simulink model "ieee_6_bus_base_case"  (R2015b)
settings: Solver=FixedStepAuto  StartTime=0.0  StopTime=25  FixedStep=Ts  RelTol=1e-3
values from neighbouring files (symbols this model uses):
  Cbase = 1/(100*pi*Xbase)    (= 1.34217357979e-05)    [ieee_6_bus.m]
  Lbase = Xbase/(100*pi)    (= 0.754903726073)    [ieee_6_bus.m]
  Ts = 1e-5    (= 1e-05)    [ieee_6_bus.m]
  Xbase = (Vbase^2)/Sbase    (= 237.16)    [ieee_6_bus.m]
undefined symbols (not defined in the file or in its folder): loadconnection, startup
libraries: powerlib x153, powerlib_meascontrol x7, sps_avr x4, simulink x1
(part 1 of 2)
settings Model: SimulationMode=accelerator  Creator=Eren  LastModifiedBy=Eren
settings SolverCC: AlgebraicLoopSolver=LineSearch

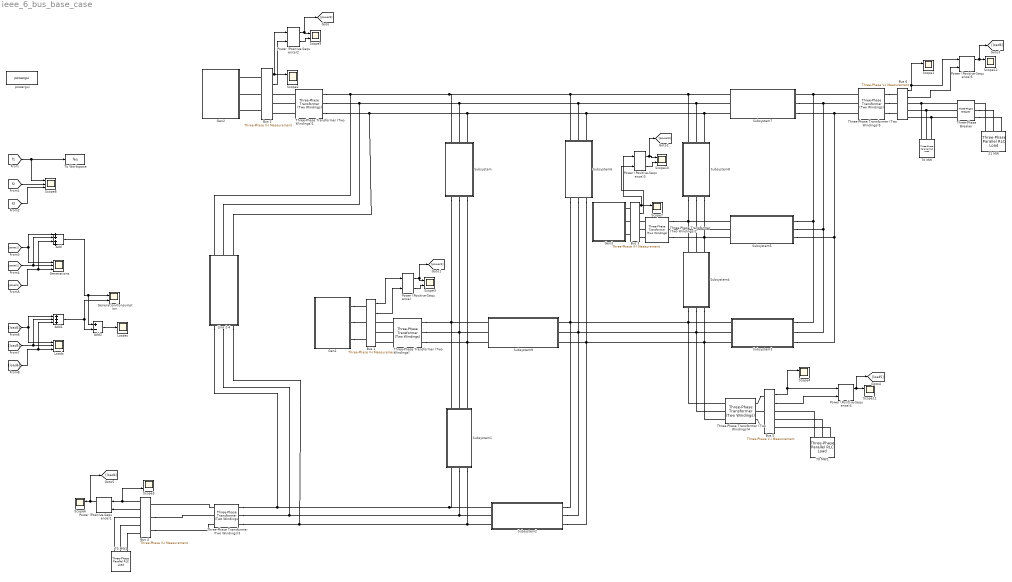
== system ieee_6_bus_base_case ==
  21 MW : powerlib/Elements/Three-Phase Parallel RLC Load  LConnTagsString=A|B|C  Configuration=Y (grounded)  NominalVoltage=690  Vabc=[1e3 1e3 1e3]  Vabcp=[1e3 1e3 1e3]  NominalFrequency=50  UnbalancedPower=off  ActivePower=21e6  InductivePower=0  CapacitivePower=0  Pabc=[10e3 9e3 11e3]  QLabc=[100 90 110]  QCabc=[100 90 110]  Pabcp=[10e3 9e3 11e3]  QLabcp=[100 90 110]  QCabcp=[100 90 110]  Measurements=None  LoadType=constant PQ
  70 MW : powerlib/Elements/Three-Phase Parallel RLC Load  LConnTagsString=A|B|C  Configuration=Y (grounded)  NominalVoltage=690  Vabc=[1e3 1e3 1e3]  Vabcp=[1e3 1e3 1e3]  NominalFrequency=50  UnbalancedPower=off  ActivePower=70e6  InductivePower=70e6  CapacitivePower=0  Pabc=[10e3 9e3 11e3]  QLabc=[100 90 110]  QCabc=[100 90 110]  Pabcp=[10e3 9e3 11e3]  QLabcp=[100 90 110]  QCabcp=[100 90 110]  Measurements=None  LoadType=constant PQ
  70 MW1 : powerlib/Elements/Three-Phase Parallel RLC Load  LConnTagsString=A|B|C  Configuration=Y (grounded)  NominalVoltage=690  Vabc=[1e3 1e3 1e3]  Vabcp=[1e3 1e3 1e3]  NominalFrequency=50  UnbalancedPower=off  ActivePower=70e6  InductivePower=70e6  CapacitivePower=0  Pabc=[10e3 9e3 11e3]  QLabc=[100 90 110]  QCabc=[100 90 110]  Pabcp=[10e3 9e3 11e3]  QLabcp=[100 90 110]  QCabcp=[100 90 110]  Measurements=None  LoadType=constant PQ
  70 MW2 : powerlib/Elements/Three-Phase Parallel RLC Load  LConnTagsString=A|B|C  Configuration=Y (grounded)  NominalVoltage=690  Vabc=[1e3 1e3 1e3]  Vabcp=[1e3 1e3 1e3]  NominalFrequency=50  UnbalancedPower=off  ActivePower=70e6  InductivePower=70e6  CapacitivePower=0  Pabc=[10e3 9e3 11e3]  QLabc=[100 90 110]  QCabc=[100 90 110]  Pabcp=[10e3 9e3 11e3]  QLabcp=[100 90 110]  QCabcp=[100 90 110]  Measurements=None  LoadType=constant PQ
  Add : Sum  Inputs=4
  Add1 : Sum  Inputs=3
  Add2 : Sum  Inputs=+-
  Bus {1..4,6} (5 alike) : powerlib/Measurements/Three-Phase V-I Measurement  VoltageMeasurement=phase-to-ground  SetLabelV=off  LabelV=Vsabc  Vpu=off  VpuLL=on  CurrentMeasurement=yes  SetLabelI=off  LabelI=Isabc  Ipu=off  Pbase=100e6  Vbase=690  OutputType=Complex  PhasorSimulation=off  PSBequivalent=0
  Bus 5 : powerlib/Measurements/Three-Phase V-I Measurement  VoltageMeasurement=phase-to-ground  SetLabelV=off  LabelV=Vsabc  Vpu=off  VpuLL=off  CurrentMeasurement=yes  SetLabelI=off  LabelI=Isabc  Ipu=off  Pbase=100e6  Vbase=690  OutputType=Complex  PhasorSimulation=off  PSBequivalent=0
  Gen1 : Subsystem
  Gen2 : Subsystem
  Gen3 : Subsystem
  Generation/Consumption : Scope  NumInputPorts=2
  Generations : Scope  NumInputPorts=3
  Line 2-4 : Subsystem
  Loads : Scope  NumInputPorts=3
  Losses : Scope
  Power (Positive-Sequence){,1..5} (6 alike) : powerlib_meascontrol/Measurements/Power (Positive-Sequence)  Freq=50  Vinit=[0, 0]  Iinit=[0, 0]  Ts=0
  Scope{1..7,9..12} (11 alike) : Scope  NumInputPorts=2
  Scope8 : Scope  NumInputPorts=3
  Subsystem : Subsystem
  Subsystem1 : Subsystem
  Subsystem2 : Subsystem
  Subsystem3 : Subsystem
  Subsystem4 : Subsystem
  Subsystem5 : Subsystem
  Subsystem6 : Subsystem
  Subsystem7 : Subsystem
  Subsystem8 : Subsystem
  Subsystem9 : Subsystem
  Three-Phase Transformer (Two Windings) : powerlib/Elements/Three-Phase Transformer (Two Windings)  Winding1Connection=Yg  Winding2Connection=Yg  CoreType=Three single-phase transformers  SetSaturation=off  Hysteresis=off  DataFile='hysteresis'  SetInitialFlux=off  Measurements=None  UNITS=pu  NominalPower=[ 250e6 , 50 ]  Winding1="[ 690 , 0.001  , 0 ]"  Winding2="[ 154e3 , 0.001  , 0 ]"  Rm=500  Lm=500  L0=0.5  Saturation=[ 0,0 ; 0.0024,1.2 ; 1.0,1.52 ]  InitialFluxes=[ 0.8 , -0.8 , 0.7 ]  MoreParameters=off  BreakLoop=off  DataType=off  TransfoNumber=1
  Three-Phase Transformer (Two Windings){1..2,4..5} (4 alike) : powerlib/Elements/Three-Phase Transformer (Two Windings)  Winding1Connection=Yg  Winding2Connection=Yg  CoreType=Three single-phase transformers  SetSaturation=off  Hysteresis=off  DataFile='hysteresis'  SetInitialFlux=off  Measurements=None  UNITS=pu  NominalPower=[ 250e6 , 50 ]  Winding1=[ 690 , 0.001 , 0 ]  Winding2="[ 154e3 , 0.001  , 0 ]"  Rm=500  Lm=500  L0=0.5  Saturation=[ 0,0 ; 0.0024,1.2 ; 1.0,1.52 ]  InitialFluxes=[ 0.8 , -0.8 , 0.7 ]  MoreParameters=off  BreakLoop=off  DataType=off  TransfoNumber=1
  Three-Phase Transformer (Two Windings)3 : powerlib/Elements/Three-Phase Transformer (Two Windings)  Winding1Connection=Yg  Winding2Connection=Yg  CoreType=Three single-phase transformers  SetSaturation=off  Hysteresis=off  DataFile='hysteresis'  SetInitialFlux=off  Measurements=None  UNITS=pu  NominalPower=[ 250e6 , 50 ]  Winding1="[ 690 , 0.001  , 0 ]"  Winding2="[ 154e3 , 0.001  , 0 ]"  Rm=500  Lm=500  L0=0.5  Saturation=[ 0,0 ; 0.0024,1.2 ; 1.0,1.52 ]  InitialFluxes=[ 0.8 , -0.8 , 0.7 ]  MoreParameters=off  BreakLoop=off  DataType=off  TransfoNumber=1
  Three-Phase Breaker : powerlib/Elements/Three-Phase Breaker  InitialState=open  SwitchA=on  SwitchB=on  SwitchC=on  SwitchTimes=loadconnection  External=off  BreakerResistance=0.01  SnubberResistance=1e6  SnubberCapacitance=inf  Measurements=None
  To Workspace : ToWorkspace  VariableName=feq  SaveFormat=Structure With Time  SampleTime=-1
      settings: Decimation=3  Save2DSignal=2-D array (concatenate along first dimension)
  powergui : powerlib/powergui  Priority=2  SimulationMode=Discrete  SolverType=Tustin  SampleTime=Ts  frequency=60  SPID=off  DisableSnubberDevices=off  DisableRonSwitches=off  DisableVfSwitches=off  SwTol=0  DisplayEquations=off  Interpol=off  ExternalGateDelay=off  methode=off  Ts=0  FunctionMessages=off  echomessages=off  HookPort=off  EnableUseOfTLC=off  x0status=blocks  frequencyindice=50  Pbase=100e6  ErrMax=1e-4  Iterations=50  UnitsV=kV  UnitsW=MW  buscounter=0  RestoreLinks=warning  ResistiveCurrentMeasurement=off  Frange=[0:2:500]  Ylog=off  Xlog=on  ShowGrid=off  save=off  variable=ZData  structure=0  ZoomFFT=on  StartTime=0.0  cycles=1  DisplayStyle=1  fundamental=60  FreqAxis=off  MaxFrequency=1000  frequencyindicesteady=1  RmsSteady=1  display=off
  wires:
  Bus 1/1 -> Power (Positive-Sequence)/1
  Bus 1/2 -> Power (Positive-Sequence)/2
  Power (Positive-Sequence)/1 -> [power1], Scope3/1
  Power (Positive-Sequence)/2 -> Scope3/2
  Bus 6/1 -> Scope1/1, Power (Positive-Sequence)5/1
  Bus 2/1 -> Power (Positive-Sequence)2/1, Scope2/1
  Bus 5/1 -> Power (Positive-Sequence)4/1, Scope4/1
  Bus 3/1 -> Power (Positive-Sequence)3/1, Scope7/1
  [f1] -> To Workspace/1, Scope8/1
  [f2] -> Scope8/2
  [f3] -> Scope8/3
  Bus 2/2 -> Power (Positive-Sequence)2/2
  Power (Positive-Sequence)2/2 -> Scope9/2
  Power (Positive-Sequence)3/1 -> [power3], Scope10/1
  Power (Positive-Sequence)3/2 -> Scope10/2
  Bus 3/2 -> Power (Positive-Sequence)3/2
  Power (Positive-Sequence)4/1 -> [load5], Scope11/1
  Bus 5/2 -> Power (Positive-Sequence)4/2
  Bus 6/2 -> Power (Positive-Sequence)5/2
  Bus 4/1 -> Scope5/2, Power (Positive-Sequence)1/1
  Bus 4/2 -> Power (Positive-Sequence)1/2
  Power (Positive-Sequence)1/1 -> [load4], Scope6/1
  Power (Positive-Sequence)2/1 -> [power2], Scope9/1
  Power (Positive-Sequence)5/1 -> [load6], Scope12/1
  [power1] -> Generations/1, Add/1
  [power2] -> Add/2, Generations/2
  [power3] -> Add/3, Generations/3
  [load4] -> Loads/1, Add1/1
  [load5] -> Add1/2, Loads/2
  [load6] -> Add1/3, Loads/3
  Add/1 -> Generation/Consumption/1, Add2/1
  Add1/1 -> Add2/2, Generation/Consumption/2
  Add2/1 -> Losses/1
  connections:
  Subsystem3/RConn1 -- Subsystem7/RConn1 -- Three-Phase Transformer (Two Windings)5/RConn1 -- Subsystem5/RConn1
  Three-Phase Transformer (Two Windings)2/RConn2 -- Subsystem8/LConn2 -- Subsystem5/LConn2 -- Subsystem4/RConn2
  Subsystem1/RConn3 -- Three-Phase Transformer (Two Windings)/RConn3 -- Subsystem/LConn3 -- Subsystem9/LConn3
  Subsystem3/LConn1 -- Three-Phase Transformer (Two Windings)4/RConn1 -- Subsystem4/LConn1 -- Subsystem9/RConn1 -- Subsystem6/LConn1 -- Subsystem2/RConn1
  Subsystem3/LConn2 -- Three-Phase Transformer (Two Windings)4/RConn2 -- Subsystem9/RConn2 -- Subsystem6/LConn2 -- Subsystem2/RConn2 -- Subsystem4/LConn2
  Subsystem3/LConn3 -- Subsystem4/LConn3 -- Subsystem9/RConn3 -- Subsystem6/LConn3 -- Subsystem2/RConn3 -- Three-Phase Transformer (Two Windings)4/RConn3
  Gen1/RConn1 -- Bus 1/LConn1
  Gen1/RConn2 -- Bus 1/LConn2
  Gen1/RConn3 -- Bus 1/LConn3
  70 MW/LConn1 -- Bus 6/RConn1 -- Three-Phase Breaker/LConn1
  70 MW/LConn2 -- Bus 6/RConn2 -- Three-Phase Breaker/LConn2
  70 MW/LConn3 -- Bus 6/RConn3 -- Three-Phase Breaker/LConn3
  Bus 2/LConn1 -- Gen2/RConn1
  Bus 2/LConn2 -- Gen2/RConn2
  Bus 2/LConn3 -- Gen2/RConn3
  Bus 3/LConn1 -- Gen3/RConn1
  Bus 3/LConn2 -- Gen3/RConn2
  Bus 3/LConn3 -- Gen3/RConn3
  Three-Phase Transformer (Two Windings)1/LConn1 -- Bus 2/RConn1
  Three-Phase Transformer (Two Windings)1/LConn2 -- Bus 2/RConn2
  Three-Phase Transformer (Two Windings)1/LConn3 -- Bus 2/RConn3
  Three-Phase Transformer (Two Windings)/LConn1 -- Bus 1/RConn1
  Three-Phase Transformer (Two Windings)/LConn2 -- Bus 1/RConn2
  Three-Phase Transformer (Two Windings)/LConn3 -- Bus 1/RConn3
  Three-Phase Transformer (Two Windings)2/LConn1 -- Bus 3/RConn1
  Three-Phase Transformer (Two Windings)2/LConn2 -- Bus 3/RConn2
  Three-Phase Transformer (Two Windings)2/LConn3 -- Bus 3/RConn3
  Three-Phase Transformer (Two Windings)5/LConn1 -- Bus 6/LConn1
  Three-Phase Transformer (Two Windings)5/LConn2 -- Bus 6/LConn2
  Three-Phase Transformer (Two Windings)5/LConn3 -- Bus 6/LConn3
  Subsystem1/RConn1 -- Three-Phase Transformer (Two Windings)/RConn1 -- Subsystem9/LConn1 -- Subsystem/LConn1
  Three-Phase Transformer (Two Windings)3/RConn2 -- Subsystem1/LConn2 -- Subsystem2/LConn2 -- Line 2-4/LConn2
  Three-Phase Transformer (Two Windings)3/RConn3 -- Subsystem2/LConn3 -- Subsystem1/LConn3 -- Line 2-4/LConn3
  Line 2-4/LConn1 -- Subsystem2/LConn1 -- Subsystem1/LConn1 -- Three-Phase Transformer (Two Windings)3/RConn1
  Three-Phase Transformer (Two Windings)5/RConn3 -- Subsystem3/RConn3 -- Subsystem5/RConn3 -- Subsystem7/RConn3
  Three-Phase Transformer (Two Windings)5/RConn2 -- Subsystem3/RConn2 -- Subsystem5/RConn2 -- Subsystem7/RConn2
  Three-Phase Transformer (Two Windings)2/RConn3 -- Subsystem4/RConn3 -- Subsystem5/LConn3 -- Subsystem8/LConn3
  Line 2-4/RConn1 -- Three-Phase Transformer (Two Windings)1/RConn1 -- Subsystem8/RConn1 -- Subsystem7/LConn1 -- Subsystem6/RConn1 -- Subsystem/RConn1
  Subsystem6/RConn3 -- Line 2-4/RConn3 -- Three-Phase Transformer (Two Windings)1/RConn3 -- Subsystem/RConn3 -- Subsystem8/RConn3 -- Subsystem7/LConn3
  Three-Phase Transformer (Two Windings)1/RConn2 -- Line 2-4/RConn2 -- Subsystem8/RConn2 -- Subsystem7/LConn2 -- Subsystem6/RConn2 -- Subsystem/RConn2
  Three-Phase Transformer (Two Windings)2/RConn1 -- Subsystem8/LConn1 -- Subsystem5/LConn1 -- Subsystem4/RConn1
  Subsystem1/RConn2 -- Three-Phase Transformer (Two Windings)/RConn2 -- Subsystem/LConn2 -- Subsystem9/LConn2
  70 MW1/LConn1 -- Bus 5/RConn1
  70 MW1/LConn2 -- Bus 5/RConn2
  70 MW1/LConn3 -- Bus 5/RConn3
  Bus 5/LConn2 -- Three-Phase Transformer (Two Windings)4/LConn2
  Bus 5/LConn1 -- Three-Phase Transformer (Two Windings)4/LConn1
  Bus 5/LConn3 -- Three-Phase Transformer (Two Windings)4/LConn3
  Bus 4/LConn2 -- Three-Phase Transformer (Two Windings)3/LConn2
  Three-Phase Transformer (Two Windings)3/LConn1 -- Bus 4/LConn1
  Bus 4/LConn3 -- Three-Phase Transformer (Two Windings)3/LConn3
  Bus 4/RConn1 -- 70 MW2/LConn1
  Bus 4/RConn2 -- 70 MW2/LConn2
  Bus 4/RConn3 -- 70 MW2/LConn3
  Three-Phase Breaker/RConn3 -- 21 MW/LConn3
  21 MW/LConn1 -- Three-Phase Breaker/RConn1
  Three-Phase Breaker/RConn2 -- 21 MW/LConn2

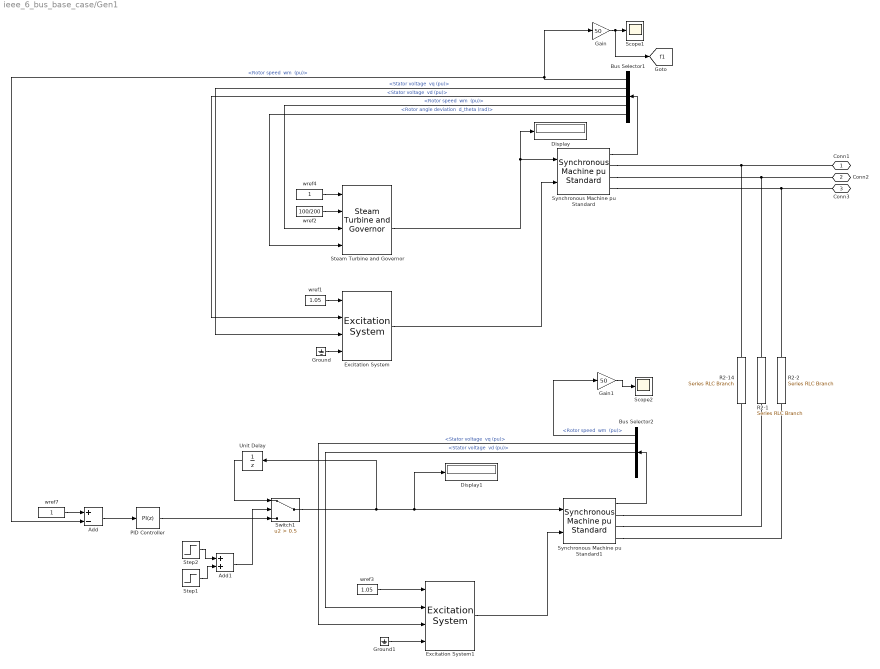
== system ieee_6_bus_base_case/Gen1 ==
  Add : Sum  Inputs=+-
  Add1 : Sum
  Bus Selector1 : BusSelector  OutputSignals="Mechanical.Rotor speed  wm  (pu),dq0 components.Stator voltage  vq (pu),dq0 components.Stator voltage  vd (pu),Mechanical.Rotor speed  wm  (pu),Mechanical.Rotor angle deviation  d_theta (rad)"
  Bus Selector2 : BusSelector  OutputSignals="Mechanical.Rotor speed  wm  (pu),dq0 components.Stator voltage  vq (pu),dq0 components.Stator voltage  vd (pu),Mechanical.Rotor speed  wm  (pu),Mechanical.Rotor angle deviation  d_theta (rad)"
  Display : Display
  Display1 : Display
  Excitation System : sps_avr/Excitation System  tr=20e-3  reg=[ 350, 0.001 ]  exc=[ 1, 0 ]  tgr=[ 0, 0 ]  damp=[ 0.001, 0.1 ]  sat=[ 0, 0 ]  lim=[ -11.5, 11.5, 0 ]  v0="[1.0  1.28]"
  Excitation System1 : sps_avr/Excitation System  tr=20e-3  reg=[ 350, 0.001 ]  exc=[ 1, 0 ]  tgr=[ 0, 0 ]  damp=[ 0.001, 0.1 ]  sat=[ 0, 0 ]  lim=[ -11.5, 11.5, 0 ]  v0="[1.0  1.28]"
  Gain : Gain  Gain=50
  Gain1 : Gain  Gain=50
  Ground : Ground
  Ground1 : Ground
  PID Controller : simulink/Continuous/PID Controller  Controller=PI  TimeDomain=Discrete-time  SampleTime=Ts  IntegratorMethod=Forward Euler  FilterMethod=Forward Euler  Form=Parallel  UseFilter=on  ControllerParametersSource=internal  P=50  I=250  D=0  N=100  InitialConditionSource=internal  InitialConditionForIntegrator=0  InitialConditionForFilter=0  ExternalReset=none  LimitOutput=on  UpperSaturationLimit=1  LowerSaturationLimit=1e-6  LinearizeAsGain=on  AntiWindupMode=none  Kb=1  TrackingMode=off  Kt=1  PParamMin=[]  PParamMax=[]  IParamMin=[]  IParamMax=[]  DParamMin=[]  DParamMax=[]  NParamMin=[]  NParamMax=[]  KbParamMin=[]  KbParamMax=[]  KtParamMin=[]  KtParamMax=[]  POutMin=[]  POutMax=[]  IOutMin=[]  IOutMax=[]  DOutMin=[]  DOutMax=[]  NOutMin=[]  NOutMax=[]  KbOutMin=[]  KbOutMax=[]  KtOutMin=[]  KtOutMax=[]  IntegratorOutMin=[]  IntegratorOutMax=[]  FilterOutMin=[]  FilterOutMax=[]  SumOutMin=[]  SumOutMax=[]  SumI1OutMin=[]  SumI1OutMax=[]  SumI2OutMin=[]  SumI2OutMax=[]  SumI3OutMin=[]  SumI3OutMax=[]  SumDOutMin=[]  SumDOutMax=[]  SaturationOutMin=[]  SaturationOutMax=[]  IntegratorContinuousStateAttributes=''  IntegratorStateMustResolveToSignalObject=off  IntegratorRTWStateStorageClass=Auto  FilterContinuousStateAttributes=''  FilterStateMustResolveToSignalObject=off  FilterRTWStateStorageClass=Auto  DifferentiatorICPrevScaledInput=0  DifferentiatorOutMin=[]  DifferentiatorOutMax=[]
  R2-1 : powerlib/Elements/Series RLC Branch  LConnTagsString=__new0  RConnTagsString=__new0  BranchType=R  Resistance=0.0000001  Inductance=0.3*Xbase  SetiL0=off  InitialCurrent=0  Capacitance=1e-6  Setx0=off  InitialVoltage=0  Measurements=None
  R2-14 : powerlib/Elements/Series RLC Branch  LConnTagsString=__new0  RConnTagsString=__new0  BranchType=R  Resistance=0.0000001  Inductance=0.3*Xbase  SetiL0=off  InitialCurrent=0  Capacitance=1e-6  Setx0=off  InitialVoltage=0  Measurements=None
  R2-2 : powerlib/Elements/Series RLC Branch  LConnTagsString=__new0  RConnTagsString=__new0  BranchType=R  Resistance=0.0000001  Inductance=0.3*Xbase  SetiL0=off  InitialCurrent=0  Capacitance=1e-6  Setx0=off  InitialVoltage=0  Measurements=None
  Scope1 : Scope
  Scope2 : Scope
  Steam Turbine and Governor : powerlib/Machines/Steam Turbine and Governor  gentype=Tandem-compound (multi-mass)  reg1="[ 1  0.05    0 ]"  reg2="[ 0.001  0.3 ]"  reg3="[ -0.1  0.1  0  4.496]"  N=1500  turb1="[ 0  10   3.3   0.5   ]"  turb2="[ 0.5   0.5   0  0 ]"  HA="[  1.5498   0.24894  0  0 ]"  KA="[  83.47  42.702  0  0 ]"  DA="[  0.3104  0.05  0  0 ]*8"  ini1=250.35/555  ini2=[0.5,-120.13]
  Step1 : Step  Time=loadconnection-1  SampleTime=Ts
  Step2 : Step  Time=startup  Before=1  After=0  SampleTime=Ts
  Switch1 : Switch  Criteria=u2 > Threshold  Threshold=0.5
  Synchronous Machine pu Standard : powerlib/Machines/Synchronous Machine pu Standard  PresetModel=No  MechanicalLoad=Mechanical power Pm  ShowDetailedParameters=on  RotorType=Round  Units=per unit standard parameters  MeasurementBus=off  NominalParameters=[200e+06 690 50]  Reactances1=[ 1.81, 0.3, 0.23, 1.76, 0.65, 0.25, 0.15 ]  Reactances2=[2.24 0.17 0.12 1.02 0.13 0.08]  dAxisTimeConstants=Short-circuit  qAxisTimeConstants=Short-circuit  TimeConstants1="[ 4.4849  0.0681  0.1  ]"  TimeConstants2=[ 8.0, 0.03, 1.0, 0.07 ]  TimeConstants3="[  4.49  0.0681  0.0513  ]"  TimeConstants4=[ 8.0, 0.03, 0.3371, 0.0295 ]  TimeConstants5=[ 1.01, 0.053, 0.1 ]  TimeConstants6=[ 1.3201, 0.023, 1.0, 0.07 ]  TimeConstants7=[0.012 0.003 0.003]  TimeConstants8=[ 1.3201, 0.0231, 0.3371, 0.0295 ]  StatorResistance=0.0000107875  Mechanical=[4 0.02056 4]  PolePairs=20  InitialConditions="[ 0  0  0  0  0  0  0  0  1 ]"  SetSaturation=off  Saturation=[0.6404,0.7127,0.8441,0.9214,0.9956,1.082,1.19,1.316,1.457;0.7,0.7698,0.8872,0.9466,0.9969,1.046,1.1,1.151,1.201]  LoadFlowParameters=[1,0,0,0,0]  TsPowergui=0  TsBlock=-1  IterativeModel=Trapezoidal non iterative  BusType=swing  Pref=0  Qref=0  Qmin=-inf  Qmax=inf  PLF=0  QLF=0
  Synchronous Machine pu Standard1 : powerlib/Machines/Synchronous Machine pu Standard  PresetModel=No  MechanicalLoad=Mechanical power Pm  ShowDetailedParameters=on  RotorType=Round  Units=per unit standard parameters  MeasurementBus=off  NominalParameters=[25e+06 690 50]  Reactances1=[ 1.81, 0.3, 0.23, 1.76, 0.65, 0.25, 0.15 ]  Reactances2=[2.24 0.17 0.12 1.02 0.13 0.08]  dAxisTimeConstants=Short-circuit  qAxisTimeConstants=Short-circuit  TimeConstants1="[ 4.4849  0.0681  0.1  ]"  TimeConstants2=[ 8.0, 0.03, 1.0, 0.07 ]  TimeConstants3="[  4.49  0.0681  0.0513  ]"  TimeConstants4=[ 8.0, 0.03, 0.3371, 0.0295 ]  TimeConstants5=[ 1.01, 0.053, 0.1 ]  TimeConstants6=[ 1.3201, 0.023, 1.0, 0.07 ]  TimeConstants7=[0.012 0.003 0.003]  TimeConstants8=[ 1.3201, 0.0231, 0.3371, 0.0295 ]  StatorResistance=0.0000107875  Mechanical=[2 0.02056 4]  PolePairs=20  InitialConditions="[ 0  0  0  0  0  0  0  0  1 ]"  SetSaturation=off  Saturation=[0.6404,0.7127,0.8441,0.9214,0.9956,1.082,1.19,1.316,1.457;0.7,0.7698,0.8872,0.9466,0.9969,1.046,1.1,1.151,1.201]  LoadFlowParameters=[1,0,0,0,0]  TsPowergui=0  TsBlock=-1  IterativeModel=Trapezoidal non iterative  BusType=swing  Pref=0  Qref=0  Qmin=-inf  Qmax=inf  PLF=0  QLF=0
  Unit Delay : UnitDelay  SampleTime=Ts
  wref1 : Constant  Value=1.05
  wref2 : Constant  Value=100/200
  wref3 : Constant  Value=1.05
  wref4 : Constant
  wref7 : Constant
  Conn1 : PMIOPort  Port=1  Side=Right
  Conn2 : PMIOPort  Port=2  Side=Right
  Conn3 : PMIOPort  Port=3  Side=Right
  tag scope: f1=global
  wires:
  Synchronous Machine pu Standard/1 -> Bus Selector1/1
  wref1/1 -> Excitation System/1
  Ground/1 -> Excitation System/4
  Excitation System/1 -> Synchronous Machine pu Standard/2
  Bus Selector1/3 -> Excitation System/2  "<Stator voltage  vd (pu)>"
  Bus Selector1/1 -> Add/2, Gain/1  "<Rotor speed  wm  (pu)>"
  Bus Selector1/2 -> Excitation System/3  "<Stator voltage  vq (pu)>"
  Gain/1 -> [f1], Scope1/1
  Bus Selector1/4 -> Steam Turbine and Governor/3  "<Rotor speed  wm  (pu)>"
  wref4/1 -> Steam Turbine and Governor/1
  Bus Selector1/5 -> Steam Turbine and Governor/4  "<Rotor angle deviation  d_theta (rad)>"
  Steam Turbine and Governor/3 -> Display/1, Synchronous Machine pu Standard/1
  wref2/1 -> Steam Turbine and Governor/2
  Synchronous Machine pu Standard1/1 -> Bus Selector2/1
  wref3/1 -> Excitation System1/1
  Ground1/1 -> Excitation System1/4
  Excitation System1/1 -> Synchronous Machine pu Standard1/2
  Bus Selector2/3 -> Excitation System1/2  "<Stator voltage  vd (pu)>"
  Bus Selector2/1 -> Gain1/1  "<Rotor speed  wm  (pu)>"
  Bus Selector2/2 -> Excitation System1/3  "<Stator voltage  vq (pu)>"
  Gain1/1 -> Scope2/1
  Switch1/1 -> Unit Delay/1, Display1/1, Synchronous Machine pu Standard1/1
  Unit Delay/1 -> Switch1/1
  wref7/1 -> Add/1
  Add/1 -> PID Controller/1
  PID Controller/1 -> Switch1/3
  Step2/1 -> Add1/1
  Step1/1 -> Add1/2
  Add1/1 -> Switch1/2
  connections:
  Synchronous Machine pu Standard/RConn3 -- R2-2/LConn1 -- Conn3/RConn1
  Synchronous Machine pu Standard/RConn2 -- R2-1/LConn1 -- Conn2/RConn1
  Synchronous Machine pu Standard/RConn1 -- R2-14/LConn1 -- Conn1/RConn1
  Synchronous Machine pu Standard1/RConn3 -- R2-2/RConn1
  Synchronous Machine pu Standard1/RConn2 -- R2-1/RConn1
  Synchronous Machine pu Standard1/RConn1 -- R2-14/RConn1

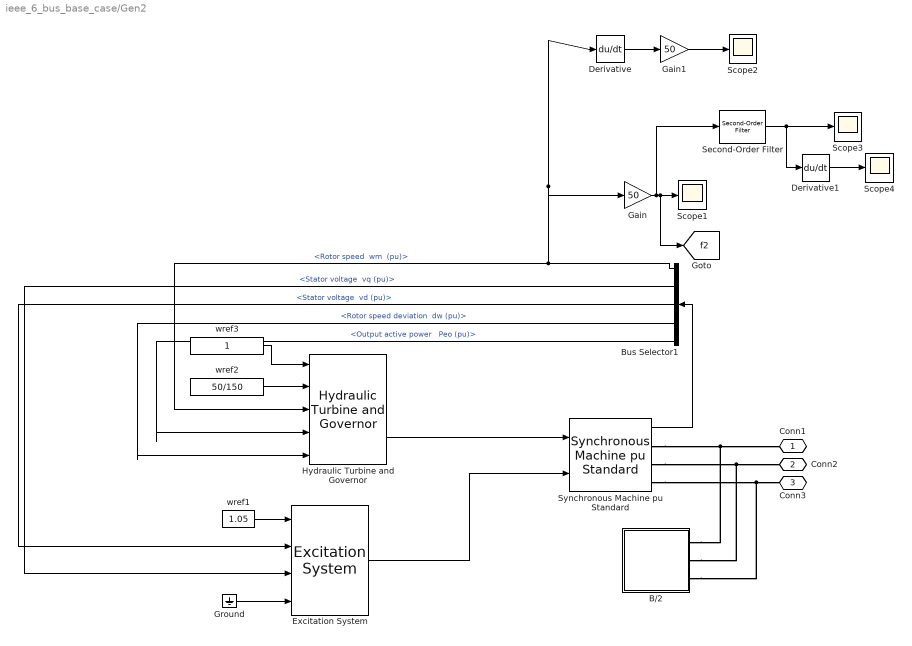
== system ieee_6_bus_base_case/Gen2 ==
  B/2 : Subsystem
  Bus Selector1 : BusSelector  OutputSignals="Mechanical.Rotor speed  wm  (pu),dq0 components.Stator voltage  vq (pu),dq0 components.Stator voltage  vd (pu),Mechanical.Rotor speed deviation  dw (pu),Output active power   Peo (pu)"
  Derivative : Derivative
  Derivative1 : Derivative
  Excitation System : sps_avr/Excitation System  tr=20e-3  reg=[ 350, 0.001 ]  exc=[ 1, 0 ]  tgr=[ 0, 0 ]  damp=[ 0.001, 0.1 ]  sat=[ 0, 0 ]  lim=[ -11.5, 11.5, 0 ]  v0="[1.0  1.28]"
  Gain : Gain  Gain=50
  Gain1 : Gain  Gain=50
  Ground : Ground
  Hydraulic Turbine and Governor : powerlib/Machines/Hydraulic Turbine and Governor  sm="[ 10/3  0.07 ]"  gate="[  0.01  0.97518  -0.1  0.1 ]"  reg="[  0.05  1.163  0.105  0  0.01  ]"  hyd="[  0  2.67  ]"  dref=0  po=1/3
  Scope{1..4} (4 alike) : Scope
  Second-Order Filter : powerlib_meascontrol/Filters/Second-Order Filter  FilterType=Lowpass  Fo=10  Zeta=0.707  Ts=Ts  Initialize=off  Vac_Init="[0,  0,  60]"  Vdc_Init=0  PlotResponse=off  FreqRange=[0, 500, 1]
  Synchronous Machine pu Standard : powerlib/Machines/Synchronous Machine pu Standard  PresetModel=No  MechanicalLoad=Mechanical power Pm  ShowDetailedParameters=on  RotorType=Round  Units=per unit standard parameters  MeasurementBus=off  NominalParameters=[150e+06 690 50]  Reactances1=[ 1.81, 0.3, 0.23, 1.76, 0.65, 0.25, 0.15 ]  Reactances2=[2.24 0.17 0.12 1.02 0.13 0.08]  dAxisTimeConstants=Short-circuit  qAxisTimeConstants=Short-circuit  TimeConstants1="[ 4.4849  0.0681  0.1  ]"  TimeConstants2=[ 8.0, 0.03, 1.0, 0.07 ]  TimeConstants3="[  4.49  0.0681  0.0513  ]"  TimeConstants4=[ 8.0, 0.03, 0.3371, 0.0295 ]  TimeConstants5=[ 1.01, 0.053, 0.1 ]  TimeConstants6=[ 1.3201, 0.023, 1.0, 0.07 ]  TimeConstants7=[0.012 0.003 0.003]  TimeConstants8=[ 1.3201, 0.0231, 0.3371, 0.0295 ]  StatorResistance=0.00000107875  Mechanical=[4 0.02056 4]  PolePairs=20  InitialConditions="[ 0  0  0  0  0  0  0  0  1 ]"  SetSaturation=off  Saturation=[0.6404,0.7127,0.8441,0.9214,0.9956,1.082,1.19,1.316,1.457;0.7,0.7698,0.8872,0.9466,0.9969,1.046,1.1,1.151,1.201]  LoadFlowParameters=[1,0,0,0,0]  TsPowergui=0  TsBlock=-1  IterativeModel=Trapezoidal non iterative  BusType=PV  Pref=50e6  Qref=0  Qmin=-inf  Qmax=inf  PLF=0  QLF=0
  wref1 : Constant  Value=1.05
  wref2 : Constant  Value=50/150
  wref3 : Constant
  Conn1 : PMIOPort  Port=1  Side=Right
  Conn2 : PMIOPort  Port=2  Side=Right
  Conn3 : PMIOPort  Port=3  Side=Right
  tag scope: f2=global
  wires:
  Derivative/1 -> Gain1/1
  Hydraulic Turbine and Governor/2 -> Synchronous Machine pu Standard/1
  Gain/1 -> Second-Order Filter/1, [f2], Scope1/1
  Bus Selector1/2 -> Excitation System/3  "<Stator voltage  vq (pu)>"
  Bus Selector1/1 -> Hydraulic Turbine and Governor/3, Gain/1, Derivative/1  "<Rotor speed  wm  (pu)>"
  Bus Selector1/3 -> Excitation System/2  "<Stator voltage  vd (pu)>"
  Excitation System/1 -> Synchronous Machine pu Standard/2
  Ground/1 -> Excitation System/4
  wref1/1 -> Excitation System/1
  Synchronous Machine pu Standard/1 -> Bus Selector1/1
  wref3/1 -> Hydraulic Turbine and Governor/1
  Bus Selector1/4 -> Hydraulic Turbine and Governor/5  "<Rotor speed deviation  dw (pu)>"
  Bus Selector1/5 -> Hydraulic Turbine and Governor/4  "<Output active power   Peo (pu)>"
  wref2/1 -> Hydraulic Turbine and Governor/2
  Second-Order Filter/1 -> Derivative1/1, Scope3/1
  Gain1/1 -> Scope2/1
  Derivative1/1 -> Scope4/1
  connections:
  Synchronous Machine pu Standard/RConn1 -- Conn1/RConn1 -- B/2/RConn1
  Synchronous Machine pu Standard/RConn2 -- Conn2/RConn1 -- B/2/RConn2
  Synchronous Machine pu Standard/RConn3 -- Conn3/RConn1 -- B/2/RConn3

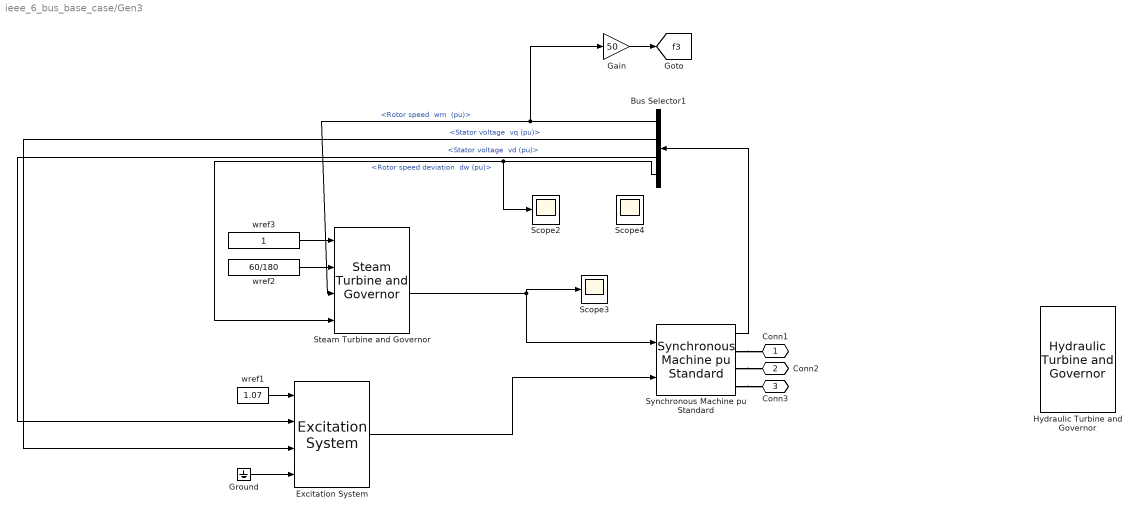
== system ieee_6_bus_base_case/Gen3 ==
  Bus Selector1 : BusSelector  OutputSignals="Mechanical.Rotor speed  wm  (pu),dq0 components.Stator voltage  vq (pu),dq0 components.Stator voltage  vd (pu),Mechanical.Rotor speed deviation  dw (pu)"
  Excitation System : sps_avr/Excitation System  tr=20e-3  reg=[ 350, 0.001 ]  exc=[ 1, 0 ]  tgr=[ 0, 0 ]  damp=[ 0.001, 0.1 ]  sat=[ 0, 0 ]  lim=[ -11.5, 11.5, 0 ]  v0="[1.0  1.28]"
  Gain : Gain  Gain=50
  Ground : Ground
  Hydraulic Turbine and Governor : powerlib/Machines/Hydraulic Turbine and Governor  sm="[ 10/3  0.07 ]"  gate="[  0.01  0.97518  -0.1  0.1 ]"  reg="[  0.05  1.163  0.105  0  0.01  ]"  hyd="[  0  2.67  ]"  dref=0  po=1/3
  Scope2 : Scope
  Scope3 : Scope
  Scope4 : Scope
  Steam Turbine and Governor : powerlib/Machines/Steam Turbine and Governor  gentype=Tandem-compound (multi-mass)  reg1="[ 1  0.05    0 ]"  reg2="[ 0.001  0.3 ]"  reg3="[ -0.1  0.1  0  4.496]"  N=1500  turb1="[ 0  10   3.3   0.5   ]"  turb2="[ 0.5   0.5   0  0 ]"  HA="[  1.5498   0.24894  0  0 ]"  KA="[  83.47  42.702  0  0 ]"  DA="[  0.3104  0.05  0  0 ]*8"  ini1=250.35/555  ini2=[0.5,-120.13]
  Synchronous Machine pu Standard : powerlib/Machines/Synchronous Machine pu Standard  PresetModel=No  MechanicalLoad=Mechanical power Pm  ShowDetailedParameters=on  RotorType=Round  Units=per unit standard parameters  MeasurementBus=off  NominalParameters=[180e+06 690 50]  Reactances1=[ 1.81, 0.3, 0.23, 1.76, 0.65, 0.25, 0.15 ]  Reactances2=[2.24 0.17 0.12 1.02 0.13 0.08]  dAxisTimeConstants=Short-circuit  qAxisTimeConstants=Short-circuit  TimeConstants1="[ 4.4849  0.0681  0.1  ]"  TimeConstants2=[ 8.0, 0.03, 1.0, 0.07 ]  TimeConstants3="[  4.49  0.0681  0.0513  ]"  TimeConstants4=[ 8.0, 0.03, 0.3371, 0.0295 ]  TimeConstants5=[ 1.01, 0.053, 0.1 ]  TimeConstants6=[ 1.3201, 0.023, 1.0, 0.07 ]  TimeConstants7=[0.012 0.003 0.003]  TimeConstants8=[ 1.3201, 0.0231, 0.3371, 0.0295 ]  StatorResistance=0.00000107875  Mechanical=[4 0.02056 4]  PolePairs=20  InitialConditions="[ 0  0  0  0  0  0  0  0  1 ]"  SetSaturation=off  Saturation=[0.6404,0.7127,0.8441,0.9214,0.9956,1.082,1.19,1.316,1.457;0.7,0.7698,0.8872,0.9466,0.9969,1.046,1.1,1.151,1.201]  LoadFlowParameters=[1,0,0,0,0]  TsPowergui=0  TsBlock=-1  IterativeModel=Trapezoidal non iterative  BusType=PV  Pref=60e6  Qref=0  Qmin=-inf  Qmax=inf  PLF=0  QLF=0
  wref1 : Constant  Value=1.07
  wref2 : Constant  Value=60/180
  wref3 : Constant
  Conn1 : PMIOPort  Port=1  Side=Right
  Conn2 : PMIOPort  Port=2  Side=Right
  Conn3 : PMIOPort  Port=3  Side=Right
  tag scope: f3=global
  wires:
  Synchronous Machine pu Standard/1 -> Bus Selector1/1
  wref1/1 -> Excitation System/1
  Ground/1 -> Excitation System/4
  Excitation System/1 -> Synchronous Machine pu Standard/2
  Bus Selector1/3 -> Excitation System/2  "<Stator voltage  vd (pu)>"
  Bus Selector1/1 -> Steam Turbine and Governor/3, Gain/1  "<Rotor speed  wm  (pu)>"
  Bus Selector1/2 -> Excitation System/3  "<Stator voltage  vq (pu)>"
  Gain/1 -> [f3]
  Steam Turbine and Governor/3 -> Synchronous Machine pu Standard/1, Scope3/1
  wref2/1 -> Steam Turbine and Governor/2
  wref3/1 -> Steam Turbine and Governor/1
  Bus Selector1/4 -> Steam Turbine and Governor/4, Scope2/1  "<Rotor speed deviation  dw (pu)>"
  connections:
  Synchronous Machine pu Standard/RConn3 -- Conn3/RConn1
  Synchronous Machine pu Standard/RConn2 -- Conn2/RConn1
  Synchronous Machine pu Standard/RConn1 -- Conn1/RConn1

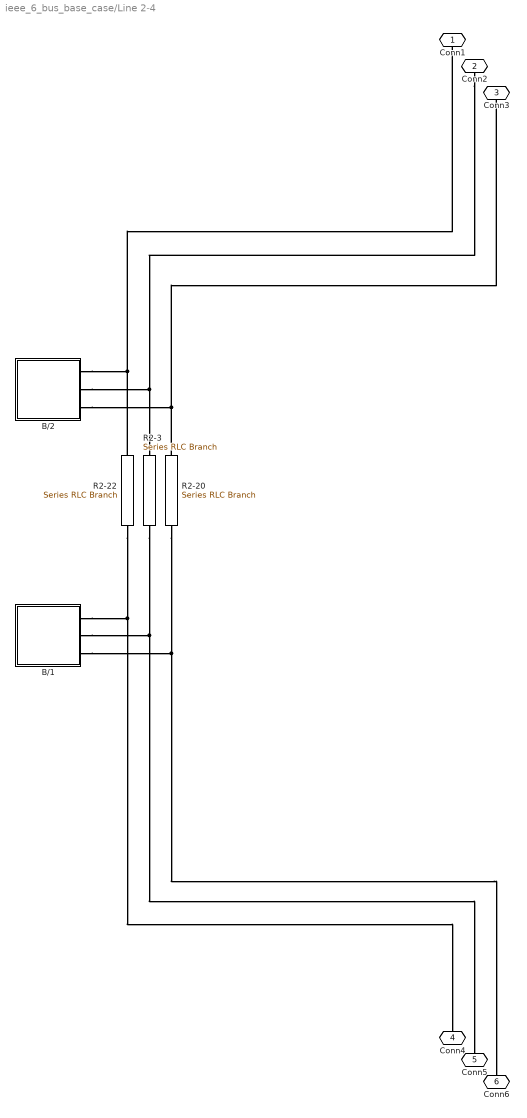
== system ieee_6_bus_base_case/Line 2-4 ==
  B/1 : Subsystem
  B/2 : Subsystem
  R2-20 : powerlib/Elements/Series RLC Branch  LConnTagsString=__new0  RConnTagsString=__new0  BranchType=RL  Resistance=0.05*Xbase  Inductance=0.1*Lbase  SetiL0=off  InitialCurrent=0  Capacitance=1e-6  Setx0=off  InitialVoltage=0  Measurements=None
  R2-22 : powerlib/Elements/Series RLC Branch  LConnTagsString=__new0  RConnTagsString=__new0  BranchType=RL  Resistance=0.05*Xbase  Inductance=0.1*Lbase  SetiL0=off  InitialCurrent=0  Capacitance=1e-6  Setx0=off  InitialVoltage=0  Measurements=None
  R2-3 : powerlib/Elements/Series RLC Branch  LConnTagsString=__new0  RConnTagsString=__new0  BranchType=RL  Resistance=0.05*Xbase  Inductance=0.1*Lbase  SetiL0=off  InitialCurrent=0  Capacitance=1e-6  Setx0=off  InitialVoltage=0  Measurements=None
  Conn1 : PMIOPort  Port=1  Side=Right
  Conn2 : PMIOPort  Port=2  Side=Right
  Conn3 : PMIOPort  Port=3  Side=Right
  Conn4 : PMIOPort  Port=4  Side=Left
  Conn5 : PMIOPort  Port=5  Side=Left
  Conn6 : PMIOPort  Port=6  Side=Left
  connections:
  R2-22/RConn1 -- B/1/RConn1 -- Conn4/RConn1
  R2-20/RConn1 -- B/1/RConn3 -- Conn6/RConn1
  Conn2/RConn1 -- B/2/RConn2 -- R2-3/LConn1
  R2-22/LConn1 -- B/2/RConn1 -- Conn1/RConn1
  R2-20/LConn1 -- B/2/RConn3 -- Conn3/RConn1
  R2-3/RConn1 -- B/1/RConn2 -- Conn5/RConn1

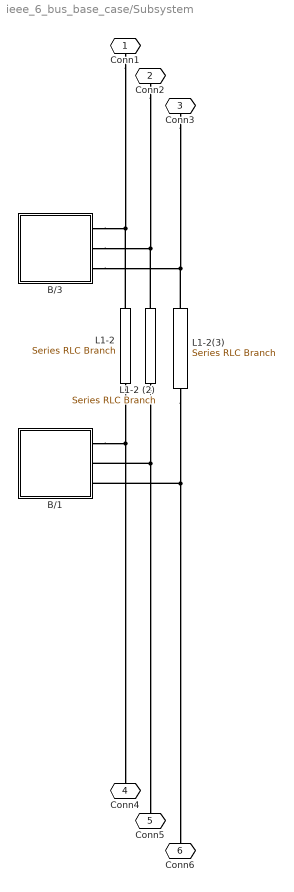
== system ieee_6_bus_base_case/Subsystem ==
  B/1 : Subsystem
  B/3 : Subsystem
  "L1-2 " : powerlib/Elements/Series RLC Branch  LConnTagsString=__new0  RConnTagsString=__new0  BranchType=RL  Resistance=0.1*Xbase  Inductance=0.2*Lbase  SetiL0=off  InitialCurrent=0  Capacitance=1e-6  Setx0=off  InitialVoltage=0  Measurements=None
  L1-2 (2) : powerlib/Elements/Series RLC Branch  LConnTagsString=__new0  RConnTagsString=__new0  BranchType=RL  Resistance=0.1*Xbase  Inductance=0.2*Lbase  SetiL0=off  InitialCurrent=0  Capacitance=1e-6  Setx0=off  InitialVoltage=0  Measurements=None
  L1-2(3) : powerlib/Elements/Series RLC Branch  LConnTagsString=__new0  RConnTagsString=__new0  BranchType=RL  Resistance=0.1*Xbase  Inductance=0.2*Lbase  SetiL0=off  InitialCurrent=0  Capacitance=1e-6  Setx0=off  InitialVoltage=0  Measurements=None
  Conn1 : PMIOPort  Port=1  Side=Right
  Conn2 : PMIOPort  Port=2  Side=Right
  Conn3 : PMIOPort  Port=3  Side=Right
  Conn4 : PMIOPort  Port=4  Side=Left
  Conn5 : PMIOPort  Port=5  Side=Left
  Conn6 : PMIOPort  Port=6  Side=Left
  connections:
  B/3/RConn1 -- Conn1/RConn1 -- "L1-2 "/LConn1
  L1-2 (2)/RConn1 -- Conn5/RConn1 -- B/1/RConn2
  "L1-2 "/RConn1 -- Conn4/RConn1 -- B/1/RConn1
  B/3/RConn3 -- Conn3/RConn1 -- L1-2(3)/LConn1
  L1-2(3)/RConn1 -- Conn6/RConn1 -- B/1/RConn3
  L1-2 (2)/LConn1 -- Conn2/RConn1 -- B/3/RConn2

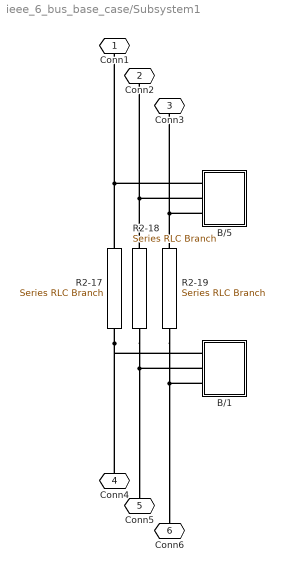
== system ieee_6_bus_base_case/Subsystem1 ==
  B/1 : Subsystem
  B/5 : Subsystem
  R2-17 : powerlib/Elements/Series RLC Branch  LConnTagsString=__new0  RConnTagsString=__new0  BranchType=RL  Resistance=0.05*Xbase  Inductance=0.2*Lbase  SetiL0=off  InitialCurrent=0  Capacitance=1e-6  Setx0=off  InitialVoltage=0  Measurements=None
  R2-18 : powerlib/Elements/Series RLC Branch  LConnTagsString=__new0  RConnTagsString=__new0  BranchType=RL  Resistance=0.05*Xbase  Inductance=0.2*Lbase  SetiL0=off  InitialCurrent=0  Capacitance=1e-6  Setx0=off  InitialVoltage=0  Measurements=None
  R2-19 : powerlib/Elements/Series RLC Branch  LConnTagsString=__new0  RConnTagsString=__new0  BranchType=RL  Resistance=0.05*Xbase  Inductance=0.2*Lbase  SetiL0=off  InitialCurrent=0  Capacitance=1e-6  Setx0=off  InitialVoltage=0  Measurements=None
  Conn1 : PMIOPort  Port=1  Side=Right
  Conn2 : PMIOPort  Port=2  Side=Right
  Conn3 : PMIOPort  Port=3  Side=Right
  Conn4 : PMIOPort  Port=4  Side=Left
  Conn5 : PMIOPort  Port=5  Side=Left
  Conn6 : PMIOPort  Port=6  Side=Left
  connections:
  R2-18/RConn1 -- Conn5/RConn1 -- B/1/RConn2
  R2-19/RConn1 -- Conn6/RConn1 -- B/1/RConn3
  R2-17/RConn1 -- Conn4/RConn1 -- B/1/RConn1
  B/5/RConn1 -- Conn1/RConn1 -- R2-17/LConn1
  R2-18/LConn1 -- Conn2/RConn1 -- B/5/RConn2
  R2-19/LConn1 -- Conn3/RConn1 -- B/5/RConn3

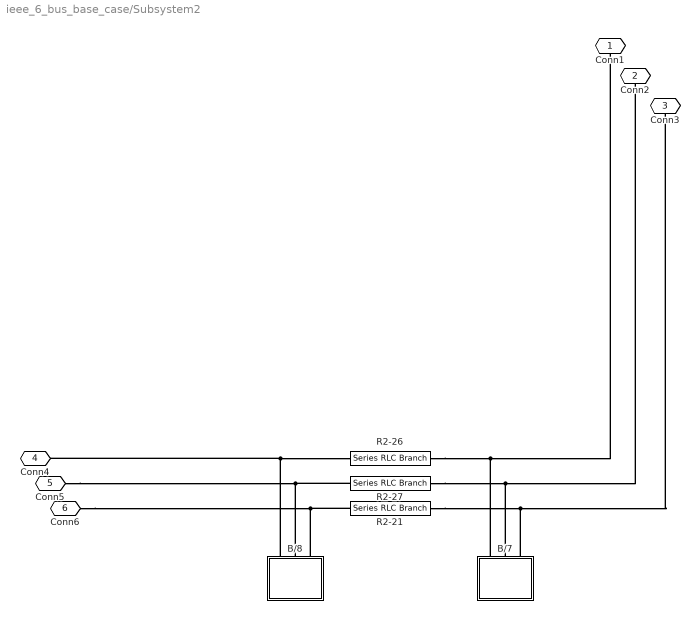
== system ieee_6_bus_base_case/Subsystem2 ==
  B/7 : Subsystem
  B/8 : Subsystem
  R2-21 : powerlib/Elements/Series RLC Branch  LConnTagsString=__new0  RConnTagsString=__new0  BranchType=RL  Resistance=0.2*Xbase  Inductance=0.4*Lbase  SetiL0=off  InitialCurrent=0  Capacitance=1e-6  Setx0=off  InitialVoltage=0  Measurements=None
  R2-26 : powerlib/Elements/Series RLC Branch  LConnTagsString=__new0  RConnTagsString=__new0  BranchType=RL  Resistance=0.2*Xbase  Inductance=0.4*Lbase  SetiL0=off  InitialCurrent=0  Capacitance=1e-6  Setx0=off  InitialVoltage=0  Measurements=None
  R2-27 : powerlib/Elements/Series RLC Branch  LConnTagsString=__new0  RConnTagsString=__new0  BranchType=RL  Resistance=0.2*Xbase  Inductance=0.4*Lbase  SetiL0=off  InitialCurrent=0  Capacitance=1e-6  Setx0=off  InitialVoltage=0  Measurements=None
  Conn1 : PMIOPort  Port=1  Side=Right
  Conn2 : PMIOPort  Port=2  Side=Right
  Conn3 : PMIOPort  Port=3  Side=Right
  Conn4 : PMIOPort  Port=4  Side=Left
  Conn5 : PMIOPort  Port=5  Side=Left
  Conn6 : PMIOPort  Port=6  Side=Left
  connections:
  B/8/RConn3 -- Conn6/RConn1 -- R2-21/RConn1
  B/8/RConn1 -- Conn4/RConn1 -- R2-26/RConn1
  R2-27/RConn1 -- Conn5/RConn1 -- B/8/RConn2
  B/7/RConn1 -- Conn1/RConn1 -- R2-26/LConn1
  B/7/RConn2 -- Conn2/RConn1 -- R2-27/LConn1
  B/7/RConn3 -- Conn3/RConn1 -- R2-21/LConn1

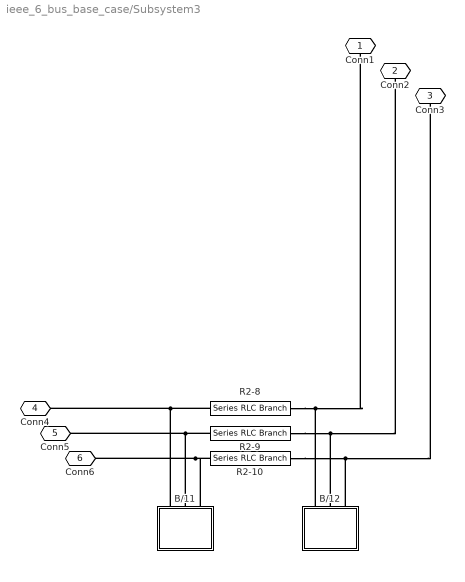
== system ieee_6_bus_base_case/Subsystem3 ==
  B/11 : Subsystem
  B/12 : Subsystem
  R2-10 : powerlib/Elements/Series RLC Branch  LConnTagsString=__new0  RConnTagsString=__new0  BranchType=RL  Resistance=0.1*Xbase  Inductance=0.3*Lbase  SetiL0=off  InitialCurrent=0  Capacitance=1e-6  Setx0=off  InitialVoltage=0  Measurements=None
  R2-8 : powerlib/Elements/Series RLC Branch  LConnTagsString=__new0  RConnTagsString=__new0  BranchType=RL  Resistance=0.1*Xbase  Inductance=0.3*Lbase  SetiL0=off  InitialCurrent=0  Capacitance=1e-6  Setx0=off  InitialVoltage=0  Measurements=None
  R2-9 : powerlib/Elements/Series RLC Branch  LConnTagsString=__new0  RConnTagsString=__new0  BranchType=RL  Resistance=0.1*Xbase  Inductance=0.3*Lbase  SetiL0=off  InitialCurrent=0  Capacitance=1e-6  Setx0=off  InitialVoltage=0  Measurements=None
  Conn1 : PMIOPort  Port=1  Side=Right
  Conn2 : PMIOPort  Port=2  Side=Right
  Conn3 : PMIOPort  Port=3  Side=Right
  Conn4 : PMIOPort  Port=4  Side=Left
  Conn5 : PMIOPort  Port=5  Side=Left
  Conn6 : PMIOPort  Port=6  Side=Left
  connections:
  R2-10/RConn1 -- Conn3/RConn1 -- B/12/RConn3
  R2-10/LConn1 -- Conn6/RConn1 -- B/11/RConn3
  R2-9/RConn1 -- Conn2/RConn1 -- B/12/RConn2
  B/12/RConn1 -- Conn1/RConn1 -- R2-8/RConn1
  R2-9/LConn1 -- Conn5/RConn1 -- B/11/RConn2
  R2-8/LConn1 -- Conn4/RConn1 -- B/11/RConn1

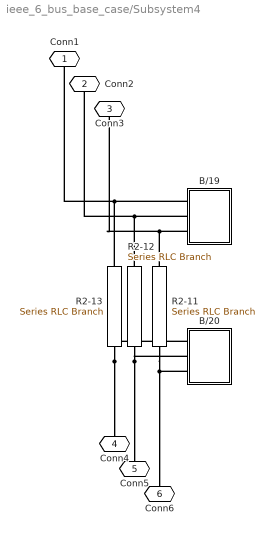
== system ieee_6_bus_base_case/Subsystem4 ==
  B/19 : Subsystem
  B/20 : Subsystem
  R2-11 : powerlib/Elements/Series RLC Branch  LConnTagsString=__new0  RConnTagsString=__new0  BranchType=RL  Resistance=0.12*Xbase  Inductance=0.26*Lbase  SetiL0=off  InitialCurrent=0  Capacitance=1e-6  Setx0=off  InitialVoltage=0  Measurements=None
  R2-12 : powerlib/Elements/Series RLC Branch  LConnTagsString=__new0  RConnTagsString=__new0  BranchType=RL  Resistance=0.12*Xbase  Inductance=0.26*Lbase  SetiL0=off  InitialCurrent=0  Capacitance=1e-6  Setx0=off  InitialVoltage=0  Measurements=None
  R2-13 : powerlib/Elements/Series RLC Branch  LConnTagsString=__new0  RConnTagsString=__new0  BranchType=RL  Resistance=0.12*Xbase  Inductance=0.26*Lbase  SetiL0=off  InitialCurrent=0  Capacitance=1e-6  Setx0=off  InitialVoltage=0  Measurements=None
  Conn1 : PMIOPort  Port=1  Side=Right
  Conn2 : PMIOPort  Port=2  Side=Right
  Conn3 : PMIOPort  Port=3  Side=Right
  Conn4 : PMIOPort  Port=4  Side=Left
  Conn5 : PMIOPort  Port=5  Side=Left
  Conn6 : PMIOPort  Port=6  Side=Left
  connections:
  R2-12/LConn1 -- Conn2/RConn1 -- B/19/RConn2
  B/20/RConn1 -- Conn4/RConn1 -- R2-13/RConn1
  B/20/RConn3 -- Conn6/RConn1 -- R2-11/RConn1
  B/19/RConn1 -- Conn1/RConn1 -- R2-13/LConn1
  B/19/RConn3 -- Conn3/RConn1 -- R2-11/LConn1
  B/20/RConn2 -- Conn5/RConn1 -- R2-12/RConn1

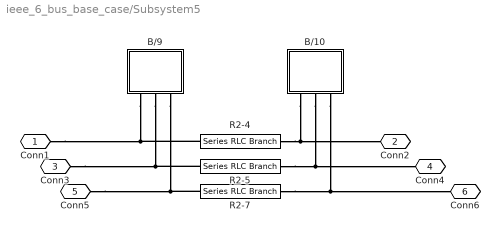
== system ieee_6_bus_base_case/Subsystem5 ==
  B/10 : Subsystem
  B/9 : Subsystem
  R2-4 : powerlib/Elements/Series RLC Branch  LConnTagsString=__new0  RConnTagsString=__new0  BranchType=RL  Resistance=0.02*Xbase  Inductance=0.1*Lbase  SetiL0=off  InitialCurrent=0  Capacitance=1e-6  Setx0=off  InitialVoltage=0  Measurements=None
  R2-5 : powerlib/Elements/Series RLC Branch  LConnTagsString=__new0  RConnTagsString=__new0  BranchType=RL  Resistance=0.02*Xbase  Inductance=0.1*Lbase  SetiL0=off  InitialCurrent=0  Capacitance=1e-6  Setx0=off  InitialVoltage=0  Measurements=None
  R2-7 : powerlib/Elements/Series RLC Branch  LConnTagsString=__new0  RConnTagsString=__new0  BranchType=RL  Resistance=0.02*Xbase  Inductance=0.1*Lbase  SetiL0=off  InitialCurrent=0  Capacitance=1e-6  Setx0=off  InitialVoltage=0  Measurements=None
  Conn1 : PMIOPort  Port=1  Side=Left
  Conn2 : PMIOPort  Port=2  Side=Right
  Conn3 : PMIOPort  Port=3  Side=Left
  Conn4 : PMIOPort  Port=4  Side=Right
  Conn5 : PMIOPort  Port=5  Side=Left
  Conn6 : PMIOPort  Port=6  Side=Right
  connections:
  R2-4/LConn1 -- Conn1/RConn1 -- B/9/RConn1
  B/9/RConn3 -- Conn5/RConn1 -- R2-7/LConn1
  R2-5/LConn1 -- Conn3/RConn1 -- B/9/RConn2
  B/10/RConn1 -- Conn2/RConn1 -- R2-4/RConn1
  R2-7/RConn1 -- Conn6/RConn1 -- B/10/RConn3
  B/10/RConn2 -- Conn4/RConn1 -- R2-5/RConn1

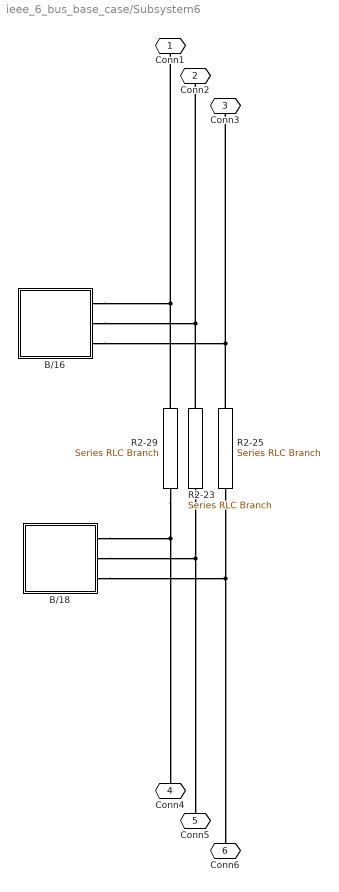
== system ieee_6_bus_base_case/Subsystem6 ==
  B/16 : Subsystem
  B/18 : Subsystem
  R2-23 : powerlib/Elements/Series RLC Branch  LConnTagsString=__new0  RConnTagsString=__new0  BranchType=RL  Resistance=0.1*Xbase  Inductance=0.3*Lbase  SetiL0=off  InitialCurrent=0  Capacitance=1e-6  Setx0=off  InitialVoltage=0  Measurements=None
  R2-25 : powerlib/Elements/Series RLC Branch  LConnTagsString=__new0  RConnTagsString=__new0  BranchType=RL  Resistance=0.1*Xbase  Inductance=0.3*Lbase  SetiL0=off  InitialCurrent=0  Capacitance=1e-6  Setx0=off  InitialVoltage=0  Measurements=None
  R2-29 : powerlib/Elements/Series RLC Branch  LConnTagsString=__new0  RConnTagsString=__new0  BranchType=RL  Resistance=0.1*Xbase  Inductance=0.3*Lbase  SetiL0=off  InitialCurrent=0  Capacitance=1e-6  Setx0=off  InitialVoltage=0  Measurements=None
  Conn1 : PMIOPort  Port=1  Side=Right
  Conn2 : PMIOPort  Port=2  Side=Right
  Conn3 : PMIOPort  Port=3  Side=Right
  Conn4 : PMIOPort  Port=4  Side=Left
  Conn5 : PMIOPort  Port=5  Side=Left
  Conn6 : PMIOPort  Port=6  Side=Left
  connections:
  R2-25/LConn1 -- Conn3/RConn1 -- B/16/RConn3
  R2-23/LConn1 -- Conn2/RConn1 -- B/16/RConn2
  B/18/RConn2 -- Conn5/RConn1 -- R2-23/RConn1
  B/18/RConn3 -- Conn6/RConn1 -- R2-25/RConn1
  R2-29/LConn1 -- Conn1/RConn1 -- B/16/RConn1
  B/18/RConn1 -- Conn4/RConn1 -- R2-29/RConn1

== system ieee_6_bus_base_case/Subsystem7 ==
  B/13 : Subsystem
  B/14 : Subsystem
  R2-28 : powerlib/Elements/Series RLC Branch  LConnTagsString=__new0  RConnTagsString=__new0  BranchType=RL  Resistance=0.07*Xbase  Inductance=0.2*Lbase  SetiL0=off  InitialCurrent=0  Capacitance=1e-6  Setx0=off  InitialVoltage=0  Measurements=None
  R2-30 : powerlib/Elements/Series RLC Branch  LConnTagsString=__new0  RConnTagsString=__new0  BranchType=RL  Resistance=0.07*Xbase  Inductance=0.2*Lbase  SetiL0=off  InitialCurrent=0  Capacitance=1e-6  Setx0=off  InitialVoltage=0  Measurements=None
  R2-6 : powerlib/Elements/Series RLC Branch  LConnTagsString=__new0  RConnTagsString=__new0  BranchType=RL  Resistance=0.07*Xbase  Inductance=0.2*Lbase  SetiL0=off  InitialCurrent=0  Capacitance=1e-6  Setx0=off  InitialVoltage=0  Measurements=None
  Conn1 : PMIOPort  Port=1  Side=Left
  Conn2 : PMIOPort  Port=2  Side=Right
  Conn3 : PMIOPort  Port=3  Side=Left
  Conn4 : PMIOPort  Port=4  Side=Right
  Conn5 : PMIOPort  Port=5  Side=Left
  Conn6 : PMIOPort  Port=6  Side=Right
  connections:
  B/14/RConn3 -- Conn5/RConn1 -- R2-30/LConn1
  B/14/RConn2 -- Conn3/RConn1 -- R2-28/LConn1
  R2-6/LConn1 -- Conn1/RConn1 -- B/14/RConn1
  R2-6/RConn1 -- Conn2/RConn1 -- B/13/RConn1
  B/13/RConn2 -- Conn4/RConn1 -- R2-28/RConn1
  R2-30/RConn1 -- Conn6/RConn1 -- B/13/RConn3

== system ieee_6_bus_base_case/Subsystem8 ==
  B/21 : Subsystem
  B/22 : Subsystem
  R2-1 : powerlib/Elements/Series RLC Branch  LConnTagsString=__new0  RConnTagsString=__new0  BranchType=RL  Resistance=0.05*Xbase  Inductance=0.25*Lbase  SetiL0=off  InitialCurrent=0  Capacitance=1e-6  Setx0=off  InitialVoltage=0  Measurements=None
  R2-2 : powerlib/Elements/Series RLC Branch  LConnTagsString=__new0  RConnTagsString=__new0  BranchType=RL  Resistance=0.05*Xbase  Inductance=0.25*Lbase  SetiL0=off  InitialCurrent=0  Capacitance=1e-6  Setx0=off  InitialVoltage=0  Measurements=None
  R2-24 : powerlib/Elements/Series RLC Branch  LConnTagsString=__new0  RConnTagsString=__new0  BranchType=RL  Resistance=0.05*Xbase  Inductance=0.25*Lbase  SetiL0=off  InitialCurrent=0  Capacitance=1e-6  Setx0=off  InitialVoltage=0  Measurements=None
  Conn1 : PMIOPort  Port=1  Side=Right
  Conn2 : PMIOPort  Port=2  Side=Right
  Conn3 : PMIOPort  Port=3  Side=Right
  Conn4 : PMIOPort  Port=4  Side=Left
  Conn5 : PMIOPort  Port=5  Side=Left
  Conn6 : PMIOPort  Port=6  Side=Left
  connections:
  B/21/RConn1 -- R2-24/LConn1 -- Conn1/RConn1
  R2-2/RConn1 -- Conn6/RConn1 -- B/22/RConn3
  B/22/RConn1 -- Conn4/RConn1 -- R2-24/RConn1
  B/21/RConn2 -- R2-1/LConn1 -- Conn2/RConn1
  B/21/RConn3 -- R2-2/LConn1 -- Conn3/RConn1
  R2-1/RConn1 -- Conn5/RConn1 -- B/22/RConn2

== system ieee_6_bus_base_case/Subsystem9 ==
  B/15 : Subsystem
  B/6 : Subsystem
  R2-14 : powerlib/Elements/Series RLC Branch  LConnTagsString=__new0  RConnTagsString=__new0  BranchType=RL  Resistance=0.08*Xbase  Inductance=0.3*Xbase  SetiL0=off  InitialCurrent=0  Capacitance=1e-6  Setx0=off  InitialVoltage=0  Measurements=None
  R2-15 : powerlib/Elements/Series RLC Branch  LConnTagsString=__new0  RConnTagsString=__new0  BranchType=RL  Resistance=0.08*Xbase  Inductance=0.3*Xbase  SetiL0=off  InitialCurrent=0  Capacitance=1e-6  Setx0=off  InitialVoltage=0  Measurements=None
  R2-16 : powerlib/Elements/Series RLC Branch  LConnTagsString=__new0  RConnTagsString=__new0  BranchType=RL  Resistance=0.08*Xbase  Inductance=0.3*Xbase  SetiL0=off  InitialCurrent=0  Capacitance=1e-6  Setx0=off  InitialVoltage=0  Measurements=None
  Conn1 : PMIOPort  Port=1  Side=Left
  Conn2 : PMIOPort  Port=2  Side=Right
  Conn3 : PMIOPort  Port=3  Side=Left
  Conn4 : PMIOPort  Port=4  Side=Right
  Conn5 : PMIOPort  Port=5  Side=Left
  Conn6 : PMIOPort  Port=6  Side=Right
  connections:
  R2-15/LConn1 -- Conn3/RConn1 -- B/15/RConn2
  B/6/RConn2 -- Conn4/RConn1 -- R2-15/RConn1
  B/6/RConn1 -- Conn2/RConn1 -- R2-14/RConn1
  B/6/RConn3 -- Conn6/RConn1 -- R2-16/RConn1
  B/15/RConn3 -- Conn5/RConn1 -- R2-16/LConn1
  B/15/RConn1 -- Conn1/RConn1 -- R2-14/LConn1

== system ieee_6_bus_base_case/Gen2/B//2 ==
  R2-1 : powerlib/Elements/Series RLC Branch  LConnTagsString=__new0  RConnTagsString=__new0  BranchType=R  Resistance=10000000000  Inductance=1e-3  SetiL0=off  InitialCurrent=0  Capacitance=1000000*Cbase  Setx0=off  InitialVoltage=0  Measurements=None
  R2-2 : powerlib/Elements/Series RLC Branch  LConnTagsString=__new0  RConnTagsString=__new0  BranchType=R  Resistance=10000000000  Inductance=1e-3  SetiL0=off  InitialCurrent=0  Capacitance=1000000*Cbase  Setx0=off  InitialVoltage=0  Measurements=None
  R2-32 : powerlib/Elements/Series RLC Branch  LConnTagsString=__new0  RConnTagsString=__new0  BranchType=R  Resistance=10000000000  Inductance=1e-3  SetiL0=off  InitialCurrent=0  Capacitance=1000000*Cbase  Setx0=off  InitialVoltage=0  Measurements=None
  Conn1 : PMIOPort  Port=1  Side=Right
  Conn2 : PMIOPort  Port=2  Side=Right
  Conn3 : PMIOPort  Port=3  Side=Right
  connections:
  R2-1/LConn1 -- Conn2/RConn1
  R2-1/RConn1 -- R2-32/RConn1 -- R2-2/RConn1
  R2-32/LConn1 -- Conn1/RConn1
  R2-2/LConn1 -- Conn3/RConn1

== system ieee_6_bus_base_case/Line 2-4/B//1 ==
  Ground : powerlib/Elements/Ground  LConnTagsString=a
  R2-1 : powerlib/Elements/Series RLC Branch  LConnTagsString=__new0  RConnTagsString=__new0  BranchType=C  Resistance=1  Inductance=1e-3  SetiL0=off  InitialCurrent=0  Capacitance=Cbase/50  Setx0=off  InitialVoltage=0  Measurements=None
  R2-2 : powerlib/Elements/Series RLC Branch  LConnTagsString=__new0  RConnTagsString=__new0  BranchType=C  Resistance=1  Inductance=1e-3  SetiL0=off  InitialCurrent=0  Capacitance=Cbase/50  Setx0=off  InitialVoltage=0  Measurements=None
  R2-32 : powerlib/Elements/Series RLC Branch  LConnTagsString=__new0  RConnTagsString=__new0  BranchType=C  Resistance=1  Inductance=1e-3  SetiL0=off  InitialCurrent=0  Capacitance=Cbase/50  Setx0=off  InitialVoltage=0  Measurements=None
  Conn1 : PMIOPort  Port=1  Side=Right
  Conn2 : PMIOPort  Port=2  Side=Right
  Conn3 : PMIOPort  Port=3  Side=Right
  connections:
  R2-32/LConn1 -- Conn1/RConn1
  R2-2/RConn1 -- R2-32/RConn1 -- Ground/LConn1 -- R2-1/RConn1
  R2-2/LConn1 -- Conn3/RConn1
  R2-1/LConn1 -- Conn2/RConn1

== system ieee_6_bus_base_case/Line 2-4/B//2 ==
  Ground : powerlib/Elements/Ground  LConnTagsString=a
  R2-1 : powerlib/Elements/Series RLC Branch  LConnTagsString=__new0  RConnTagsString=__new0  BranchType=C  Resistance=1  Inductance=1e-3  SetiL0=off  InitialCurrent=0  Capacitance=Cbase/50  Setx0=off  InitialVoltage=0  Measurements=None
  R2-2 : powerlib/Elements/Series RLC Branch  LConnTagsString=__new0  RConnTagsString=__new0  BranchType=C  Resistance=1  Inductance=1e-3  SetiL0=off  InitialCurrent=0  Capacitance=Cbase/50  Setx0=off  InitialVoltage=0  Measurements=None
  R2-32 : powerlib/Elements/Series RLC Branch  LConnTagsString=__new0  RConnTagsString=__new0  BranchType=C  Resistance=1  Inductance=1e-3  SetiL0=off  InitialCurrent=0  Capacitance=Cbase/50  Setx0=off  InitialVoltage=0  Measurements=None
  Conn1 : PMIOPort  Port=1  Side=Right
  Conn2 : PMIOPort  Port=2  Side=Right
  Conn3 : PMIOPort  Port=3  Side=Right
  connections:
  R2-1/LConn1 -- Conn2/RConn1
  R2-2/LConn1 -- Conn3/RConn1
  Ground/LConn1 -- R2-2/RConn1 -- R2-1/RConn1 -- R2-32/RConn1
  R2-32/LConn1 -- Conn1/RConn1

== system ieee_6_bus_base_case/Subsystem/B//1 ==
  C1 : powerlib/Elements/Series RLC Branch  LConnTagsString=__new0  RConnTagsString=__new0  BranchType=C  Resistance=1  Inductance=1e-3  SetiL0=off  InitialCurrent=0  Capacitance=Cbase/25  Setx0=off  InitialVoltage=0  Measurements=None
  C2 : powerlib/Elements/Series RLC Branch  LConnTagsString=__new0  RConnTagsString=__new0  BranchType=C  Resistance=1  Inductance=1e-3  SetiL0=off  InitialCurrent=0  Capacitance=Cbase/25  Setx0=off  InitialVoltage=0  Measurements=None
  C3 : powerlib/Elements/Series RLC Branch  LConnTagsString=__new0  RConnTagsString=__new0  BranchType=C  Resistance=1  Inductance=1e-3  SetiL0=off  InitialCurrent=0  Capacitance=Cbase/25  Setx0=off  InitialVoltage=0  Measurements=None
  Ground : powerlib/Elements/Ground  LConnTagsString=a
  Conn1 : PMIOPort  Port=1  Side=Right
  Conn2 : PMIOPort  Port=2  Side=Right
  Conn3 : PMIOPort  Port=3  Side=Right
  connections:
  C1/LConn1 -- Conn1/RConn1
  C3/RConn1 -- Ground/LConn1 -- C1/RConn1 -- C2/RConn1
  C3/LConn1 -- Conn3/RConn1
  C2/LConn1 -- Conn2/RConn1

== system ieee_6_bus_base_case/Subsystem/B//3 ==
  C1 : powerlib/Elements/Series RLC Branch  LConnTagsString=__new0  RConnTagsString=__new0  BranchType=C  Resistance=1  Inductance=1e-3  SetiL0=off  InitialCurrent=0  Capacitance=Cbase/25  Setx0=off  InitialVoltage=0  Measurements=None
  C2 : powerlib/Elements/Series RLC Branch  LConnTagsString=__new0  RConnTagsString=__new0  BranchType=C  Resistance=1  Inductance=1e-3  SetiL0=off  InitialCurrent=0  Capacitance=Cbase/25  Setx0=off  InitialVoltage=0  Measurements=None
  C3 : powerlib/Elements/Series RLC Branch  LConnTagsString=__new0  RConnTagsString=__new0  BranchType=C  Resistance=1  Inductance=1e-3  SetiL0=off  InitialCurrent=0  Capacitance=Cbase/25  Setx0=off  InitialVoltage=0  Measurements=None
  Ground : powerlib/Elements/Ground  LConnTagsString=a
  Conn1 : PMIOPort  Port=1  Side=Right
  Conn2 : PMIOPort  Port=2  Side=Right
  Conn3 : PMIOPort  Port=3  Side=Right
  connections:
  C2/LConn1 -- Conn2/RConn1
  C3/LConn1 -- Conn3/RConn1
  C1/RConn1 -- C3/RConn1 -- C2/RConn1 -- Ground/LConn1
  C1/LConn1 -- Conn1/RConn1

== system ieee_6_bus_base_case/Subsystem1/B//1 ==
  Ground : powerlib/Elements/Ground  LConnTagsString=a
  R2-1 : powerlib/Elements/Series RLC Branch  LConnTagsString=__new0  RConnTagsString=__new0  BranchType=C  Resistance=1  Inductance=1e-3  SetiL0=off  InitialCurrent=0  Capacitance=Cbase/25  Setx0=off  InitialVoltage=0  Measurements=None
  R2-2 : powerlib/Elements/Series RLC Branch  LConnTagsString=__new0  RConnTagsString=__new0  BranchType=C  Resistance=1  Inductance=1e-3  SetiL0=off  InitialCurrent=0  Capacitance=Cbase/25  Setx0=off  InitialVoltage=0  Measurements=None
  R2-32 : powerlib/Elements/Series RLC Branch  LConnTagsString=__new0  RConnTagsString=__new0  BranchType=C  Resistance=1  Inductance=1e-3  SetiL0=off  InitialCurrent=0  Capacitance=Cbase/25  Setx0=off  InitialVoltage=0  Measurements=None
  Conn1 : PMIOPort  Port=1  Side=Right
  Conn2 : PMIOPort  Port=2  Side=Right
  Conn3 : PMIOPort  Port=3  Side=Right
  connections:
  R2-32/LConn1 -- Conn1/RConn1
  R2-2/RConn1 -- Ground/LConn1 -- R2-32/RConn1 -- R2-1/RConn1
  R2-2/LConn1 -- Conn3/RConn1
  R2-1/LConn1 -- Conn2/RConn1
